simulink model "BMS2"  (R2021a)
settings: Solver=VariableStepAuto  StartTime=0.0  StopTime=10.0  RelTol=1e-3
undefined symbols (not defined in the file): Ion, Lithium
libraries: spsIdealSwitchLib x4, spsBatteryLib x1, spsDCVoltageSourceLib x1, spsSeriesRLCLoadLib x1, spspowerguiLib x1
settings Model: Creator=msipc  LastModifiedBy=msipc

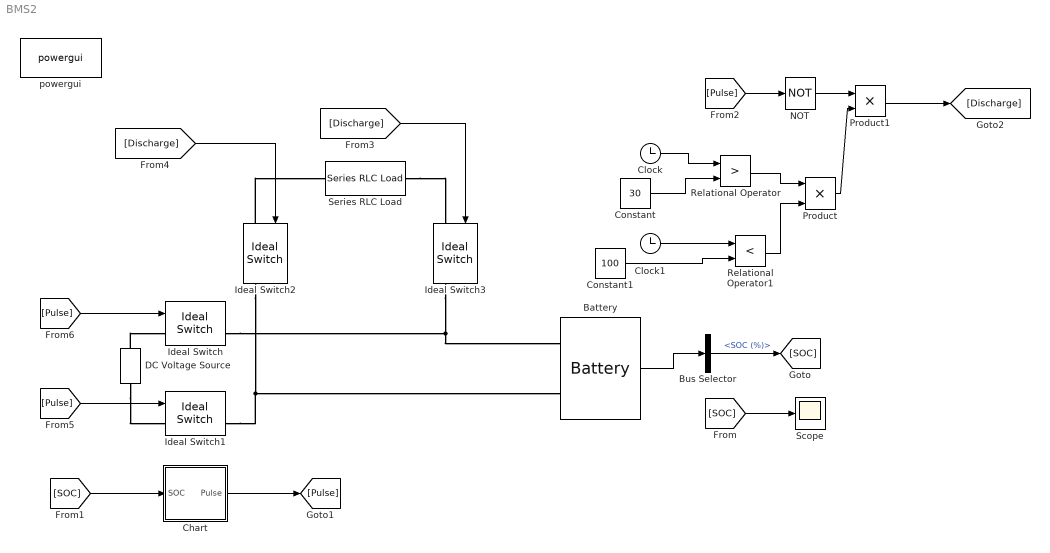
== system BMS2 ==
  Battery : spsBatteryLib/Battery  BatType=Lithium-Ion  ShowTempParam=off  ThermalPreset=no  ShowAgeParam=off  NomV=46.8  NomQ=5.4  SOC=50  Batt_Tr=1  PresetModel=on  MaxQ=5.4  MinV=35.1  FullV=54.4746  Dis_rate=2.3478  R=0.086667  Normal_OP=4.8835  expZone="[50.5621     0.265304]"  current=[6.5 13 32.5]  Units=Time  Tci=20  NomT=20  T2=-30  MaxQ2=4.8  FullV2=7.1  Normal_OP2=5.655  expZone2="[6.58           1]"  Rca=0.6  ti=2000  Dp=0  Neq0=0  Tsim=1e6  Ta1=25  Qeol=5.4*0.9  Reol=0.013333*1.2  Char_age=[2.3478, 3]  Dis_age=[2.3478, 10]  N1=1500  N2=10500  N3=1000  N4=1400  Ta2=45  N5=950
  Bus Selector : BusSelector  OutputSignals=SOC (%)
  Chart : Stateflow chart  TreatAsAtomicUnit=on
  Clock : Clock
  Clock1 : Clock
  Constant : Constant  Value=30
  Constant1 : Constant  Value=100
  DC Voltage Source : spsDCVoltageSourceLib/DC Voltage Source  Amplitude=100  Measurements=None
  Ideal Switch{,1..3} (4 alike) : spsIdealSwitchLib/Ideal Switch  Ron=0.001  Lon=0  IC=0  Rs=1e5  Cs=inf  Measurements=on
  NOT : Logic  Operator=NOT  IconShape=distinctive  AllPortsSameDT=off  OutDataTypeStr=boolean
  Product : Product  Inputs=3
  Product1 : Product
  Relational Operator : RelationalOperator  Operator=>  OutDataTypeStr=boolean  RndMeth=Simplest
  Relational Operator1 : RelationalOperator  Operator=<  OutDataTypeStr=boolean  RndMeth=Simplest
  Scope : Scope
  Series RLC Load : spsSeriesRLCLoadLib/Series RLC Load  LConnTagsString=a  RConnTagsString=__new0  NominalVoltage=10  NominalFrequency=60  ActivePower=1000  InductivePower=0  CapacitivePower=0  Setx0=off  InitialVoltage=0  SetiL0=off  InitialCurrent=0  Measurements=None  LoadType=constant Z
  powergui : spspowerguiLib/powergui  Priority=1  SimulationMode=Continuous  SampleTime=50e-6  frequency=60  Iterations=50  frequencyindice=0  Pbase=100e6  ErrMax=1e-4  UnitsV=kV  UnitsW=MW  buscounter=0  FunctionMessages=off  echomessages=off  EnableUseOfTLC=off  CurrentSourceSwitches=off  DisableSnubberDevices=off  DisableRonSwitches=off  DisableVfSwitches=off  DisplayEquations=off  AutomaticDiscreteSolvers=off  SolverType=Tustin/Backward Euler (TBE)  Interpol=off  ExternalGateDelay=off  methode=off  Ts=100  x0status=blocks  SPID=on  SwTol=0  HookPort=off  NonlinearTolerance=1e-4  nMaxIteration=100  ContinueOnMaxIteration=off  RestoreLinks=warning  ResistiveCurrentMeasurement=off  Frange=[0:2:500]  Ylog=off  Xlog=on  ShowGrid=off  save=off  variable=ZData  structure=0  ZoomFFT=off  StartTime=0.0  cycles=1  DisplayStyle=1  fundamental=60  FreqAxis=off  MaxFrequency=1000  frequencyindicesteady=1  RmsSteady=1  display=off
  wires:
  Battery/1 -> Bus Selector/1
  Bus Selector/1 -> [SOC]  "<SOC (%)>"
  [SOC] -> Scope/1
  [SOC] -> Chart/1(SOC)
  Chart/1(Pulse) -> [Pulse]
  [Pulse] -> NOT/1
  Constant/1 -> Relational Operator/2
  Clock/1 -> Relational Operator/1
  Constant1/1 -> Relational Operator1/2
  Clock1/1 -> Relational Operator1/1
  Relational Operator/1 -> Product/1
  Relational Operator1/1 -> Product/3
  NOT/1 -> Product1/1
  Product/1 -> Product1/2
  Product1/1 -> [Discharge]
  [Discharge] -> Ideal Switch2/1
  [Discharge] -> Ideal Switch3/1
  [Pulse] -> Ideal Switch1/1
  [Pulse] -> Ideal Switch/1
  connections:
  DC Voltage Source/RConn1 -- Ideal Switch1/LConn1
  DC Voltage Source/LConn1 -- Ideal Switch/LConn1
  Ideal Switch/RConn1 -- Ideal Switch3/RConn1 -- Battery/LConn2
  Ideal Switch1/RConn1 -- Ideal Switch2/RConn1 -- Battery/LConn1
  Ideal Switch2/LConn1 -- Series RLC Load/LConn1
  Series RLC Load/RConn1 -- Ideal Switch3/LConn1

== stateflow chart BMS2/Chart ==
  state Charge
    entry:Pulse=1
  state Discharge
    entry:Pulse = 0
  (default) -> Charge
  Charge -> Discharge : [SOC>75]
  Discharge -> Charge : [SOC<40]
  data: SOC input; Pulse output
